simulink model "MPC_mobile_base_KIN_IPOPT"  (R2018b)
settings: Solver=ode4  StartTime=0.0  StopTime=inf  FixedStep=Tsample  RelTol=1e-3
values from neighbouring files (symbols this model uses):
  N = 10    [STEP.m]    (also in WS.mat = 20; solver_NLP.m = evalin('base', 'N'); solver_NLP1.m = evalin('base', 'N'); traiettoria2.m = 20)
  T = 0.2    [STEP.m]    (also in WS.mat = 0.25; traiettoria2.m = 0.25; traiettoria3.m = 0.25; traiettoria4.m)
  Tsample = 0.01    [STEP.m]    (also in WS.mat; traiettoria2.m; traiettoria3.m; traiettoria4.m)
  xd = [linspace(0,5,length(tt));0.5*ones(size(tt));zeros(size(tt))]    [STEP.m]    (also in WS.mat = [0 0 0 0 0 0.000163624617374 0.0189659089948 3.10328963012e-; traiettoria2.m = [x;y+ones(size(y))*0;th]; traiettoria3.m = [x;y+ones(size(y))*0.3;th]; traiettoria4.m = [x;y+ones(size(y))*0;th])
undefined symbols (not defined in the file or in its folder): DiscIntNeverNeededParam
libraries: simulink x1, templibrary x1
settings Model: EnablePacing=on  Creator=RaffaelePC  LastModifiedBy=francesco
settings DebuggingCC: UnderSpecifiedDimensionMsg=warning

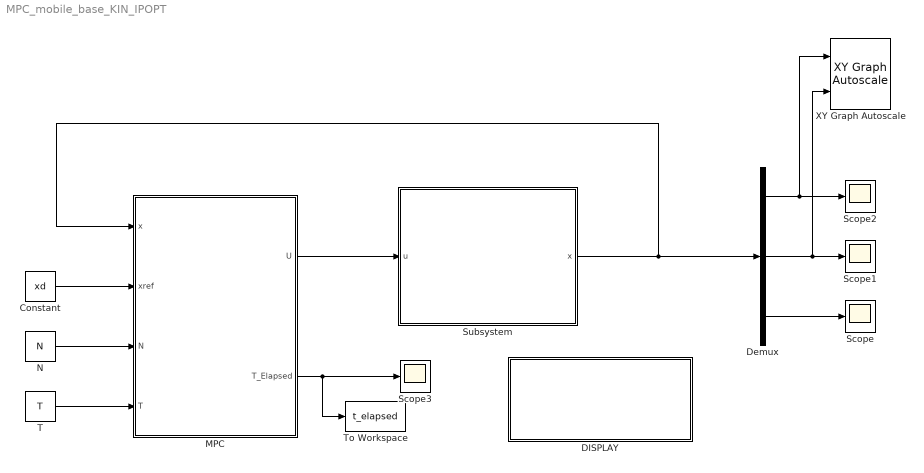
== system MPC_mobile_base_KIN_IPOPT ==
  Constant : Constant  Value=xd
  DISPLAY : Subsystem
  Demux : Demux  Outputs=3
  MPC : Subsystem
      mask Display: fprintf('MPC CONTROLLER')
  N : Constant  Value=N
  Scope{,1..3} (4 alike) : Scope
  Subsystem : Subsystem
      mask Display: disp('{\bf\fontsize{10}KINEMATIC SYSTEM}', 'texmode','on');
  T : Constant  Value=T
  To Workspace : ToWorkspace  VariableName=t_elapsed  SampleTime=T
      settings: Save2DSignal=2-D array (concatenate along first dimension)
  XY Graph Autoscale : templibrary/XY Graph  Autoscale  xmin=-1  xmax=1  ymin=-1  ymax=1  st=-1
  wires:
  N/1 -> MPC/3(N)
  T/1 -> MPC/4(T)
  Constant/1 -> MPC/2(xref)
  Subsystem/1(x) -> Demux/1, MPC/1(x)
  Demux/3 -> Scope/1
  MPC/2(T_Elapsed) -> To Workspace/1, Scope3/1
  MPC/1(U) -> Subsystem/1(u)
  Demux/2 -> XY Graph Autoscale/2, Scope1/1
  Demux/1 -> XY Graph Autoscale/1, Scope2/1

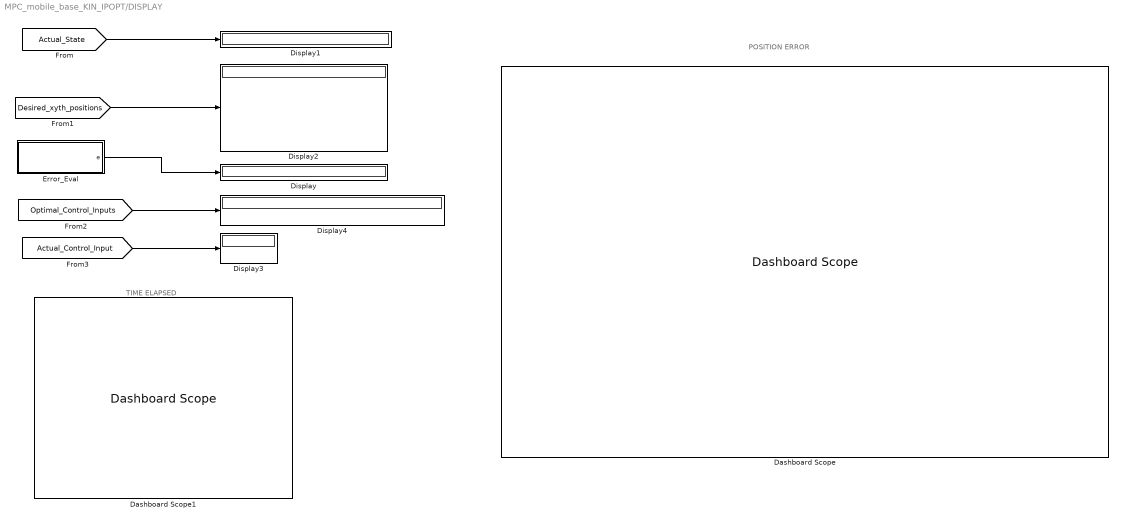
== system MPC_mobile_base_KIN_IPOPT/DISPLAY ==
  note: POSITION ERROR
  note: TIME ELAPSED
  Dashboard Scope : DashboardScope  WebBlockId=507  Ymin=-0.5  Ymax=0.5
  Dashboard Scope1 : DashboardScope  WebBlockId=516  Ymin=0  Ymax=1
  Display{,1..4} (5 alike) : Display
  "Error_Eval " : Subsystem
  wires:
  [Optimal_Control_Inputs] -> Display4/1
  [Desired_xyth_positions] -> Display2/1
  [Actual_Control_Input] -> Display3/1
  [Actual_State] -> Display1/1
  "Error_Eval "/1(e) -> Display/1

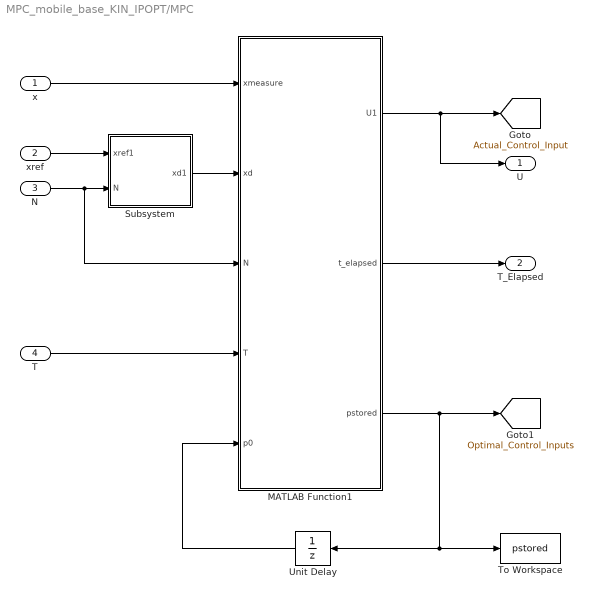
== system MPC_mobile_base_KIN_IPOPT/MPC ==
  x : Inport
  xref : Inport  Port=2
  N : Inport  Port=3
  T : Inport  Port=4
  MATLAB Function1 : MATLAB Function  TreatAsAtomicUnit=on
  Subsystem : Subsystem
  To Workspace : ToWorkspace  VariableName=pstored  SampleTime=-1
      settings: Save2DSignal=2-D array (concatenate along first dimension)
  Unit Delay : UnitDelay  InitialCondition=[0 0 0 0 0 0 0].'  SampleTime=T
  U : Outport
  T_Elapsed : Outport  Port=2
  tag scope: Actual_Control_Input=global, Optimal_Control_Inputs=global
  wires:
  Subsystem/1(xd1) -> MATLAB Function1/2(xd)
  MATLAB Function1/1(U1) -> U/1, [Actual_Control_Input]
  MATLAB Function1/3(pstored) -> To Workspace/1, Unit Delay/1, [Optimal_Control_Inputs]
  Unit Delay/1 -> MATLAB Function1/5(p0)
  xref/1 -> Subsystem/1(xref1)
  x/1 -> MATLAB Function1/1(xmeasure)
  N/1 -> MATLAB Function1/3(N), Subsystem/2(N)
  T/1 -> MATLAB Function1/4(T)
  MATLAB Function1/2(t_elapsed) -> T_Elapsed/1

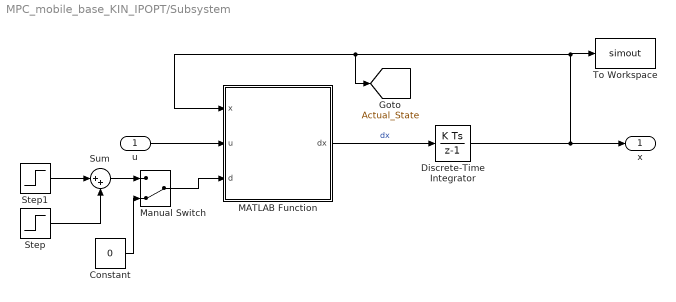
== system MPC_mobile_base_KIN_IPOPT/Subsystem ==
  u : Inport
  Constant : Constant  Value=0
  Discrete-Time Integrator : DiscreteIntegrator  InitialCondition=[0 0 0]  SampleTime=Tsample  ICPrevOutput=DiscIntNeverNeededParam  ICPrevScaledInput=DiscIntNeverNeededParam
  MATLAB Function : MATLAB Function  TreatAsAtomicUnit=on
  Manual Switch : ManualSwitch  CurrentSetting=0
  Step : Step  Time=100  SampleTime=Tsample
  Step1 : Step  Time=104  After=-1  SampleTime=Tsample
  Sum : Sum  Inputs=|++
  To Workspace : ToWorkspace  VariableName=simout  SaveFormat=Timeseries  SampleTime=Tsample
  x : Outport
  tag scope: Actual_State=global
  wires:
  u/1 -> MATLAB Function/2(u)
  MATLAB Function/1(dx) -> Discrete-Time Integrator/1  "dx"
  Discrete-Time Integrator/1 -> [Actual_State], MATLAB Function/1(x), To Workspace/1, x/1
  Step1/1 -> Sum/1
  Step/1 -> Sum/2
  Sum/1 -> Manual Switch/1
  Manual Switch/1 -> MATLAB Function/3(d)
  Constant/1 -> Manual Switch/2

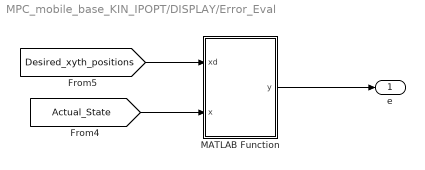
== system MPC_mobile_base_KIN_IPOPT/DISPLAY/Error_Eval  ==
  MATLAB Function : MATLAB Function  TreatAsAtomicUnit=on
  e : Outport
  wires:
  MATLAB Function/1(y) -> e/1
  [Desired_xyth_positions] -> MATLAB Function/1(xd)
  [Actual_State] -> MATLAB Function/2(x)

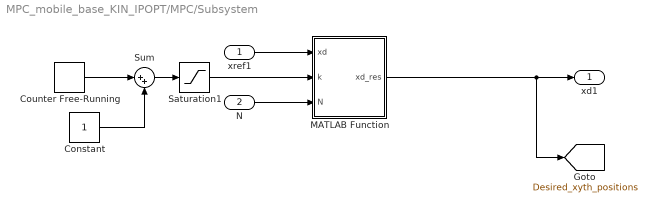
== system MPC_mobile_base_KIN_IPOPT/MPC/Subsystem ==
  xref1 : Inport
  N : Inport  Port=2
  Constant : Constant
  Counter Free-Running : simulink/Sources/Counter Free-Running  NumBits=12  tsamp=T
  MATLAB Function : MATLAB Function  TreatAsAtomicUnit=on
  Saturation1 : Saturate  UpperLimit=size(xd,2)
  Sum : Sum  Inputs=|++
  xd1 : Outport
  tag scope: Desired_xyth_positions=global
  wires:
  MATLAB Function/1(xd_res) -> [Desired_xyth_positions], xd1/1
  N/1 -> MATLAB Function/3(N)
  xref1/1 -> MATLAB Function/1(xd)
  Constant/1 -> Sum/2
  Counter Free-Running/1 -> Sum/1
  Sum/1 -> Saturation1/1
  Saturation1/1 -> MATLAB Function/2(k)

== matlab function MPC_mobile_base_KIN_IPOPT/MPC/Subsystem/MATLAB Function ==
  settings: updateMethod=DISCRETE  sampleTime=T
  data: xd input; xd_res output size=[3 N+1]; k input; N input
function xd_res   = fcn(xd,k,N)

if size(xd,2)-k>=N
h=xd(:,k:k+N);
xd_res=h;

      
else
h=[xd(:,k:end) xd(:,end)*ones(1,N-(size(xd,2)-k))];
xd_res = h;

end

== matlab function MPC_mobile_base_KIN_IPOPT/MPC/MATLAB Function1 ==
  settings: updateMethod=DISCRETE  sampleTime=T
  data: xmeasure input size=3; U1 output size=[2 1]; t_elapsed output double size=[1]; xd input; N input; T input; p0 input size=[size(p_0)]; pstored output double size=[size(p_0)] [..20]
function [U1,t_elapsed,pstored] = MPC(xmeasure,xd,N,T,p0)

coder.extrinsic('tic')
coder.extrinsic('toc')
coder.extrinsic('MPCSOLVER_KIN');

U1=zeros(2,1);

xNed=zeros(2,3);
V=0;

xN=zeros(1,3);

t_elapsed=0;

t_start=tic;

U=zeros(2,1);
xs=xd;

pstored=p0;

    %% dati solutore


% options = optimset('Display','off',...
%                 'TolFun', 1e-6,...
%                 'MaxIter', 10000,...
%                 'Algorithm', 'active-set',...
%                 'FinDiffType', 'forward',...
%                 'RelLineSrchBnd', [],...
%                 'RelLineSrchBndDuration', 1,...
%                 'TolConSQP', 1e-6);

%% MPC ALGORITHM 

x0=xmeasure;
t0=0;


   

    [u_new, pnew] = MPCSOLVER_KIN(N, x0, p0, T, xs, xd);

%   [u_new, V] = solveOptimalControlProblem ...
%         (@runningcosts, @terminalcosts, @constraints, @terminalconstraints, ...
%         @linearconstraints, @system, N, t0, x0, u0, T, xs, xd);
     
    pstored=pnew;
    U1=u_new;
    
    
t_elapsed=toc(t_start);



end

== matlab function MPC_mobile_base_KIN_IPOPT/DISPLAY/Error_Eval /MATLAB Function ==
  settings: updateMethod=DISCRETE  sampleTime=T
  data: xd input; y output size=[3 1]; x input
function y = fcn(xd,x)

h = [xd(1,1)-x(1);xd(1,2)-x(2);xd(1,3)-x(3)];
y=h;

== matlab function MPC_mobile_base_KIN_IPOPT/Subsystem/MATLAB Function ==
  settings: updateMethod=DISCRETE  sampleTime=Tsample
  data: x input; dx output; u input size=[2 1]; d input
function dx = sys_dynamics(x,u,d)
dx=zeros(1,3);
dx(1,1)=u(1,1)*cos(x(3))+d;
dx(1,2)=u(1,1)*sin(x(3))+d;
dx(1,3)=u(2,1)-0.1*d;

end
